simulink model "OFDM_Tx_Rx_fixed_point"  (R2020a)
settings: Solver=FixedStepDiscrete  StartTime=0.0  StopTime=inf  RelTol=1e-3
PostLoadFcn:
  | run ./scripts/filter_setup;
InitFcn:
  | % Set parameters
  | fs = 1e6;
  | 
  | % Load all required variables
  | load('variables/read_addr_data');
  | load('variables/read_addr_cp');
  | load('variables/read_addr_pream');
  | load('variables/read_addr_rx');
  | load('variables/pilot');
  | load('variables/sc_index');
  | load('variables/LTSfreq');
  | load('variables/STSfreq');
  | load('variables/LTSread');
  | load('variables/STSread');
undefined symbols (not defined in the file): CIC_fine_Rx, CIC_fine_Tx
libraries: dspmlti4 x7, OFDM_Rx x1, OFDM_Tx x1, dspobslib x1
settings Model: SimulationMode=accelerator  Creator=njb13206  LastModifiedBy=LDM
settings OptimizationCC: BlockReduction=off  ConditionallyExecuteInputs=off  DefaultParameterBehavior=Inlined
settings DebuggingCC: AlgebraicLoopMsg=error  IntegerOverflowMsg=none  ParameterPrecisionLossMsg=none  IntegerSaturationMsg=none
settings HardwareCC: ProdBitPerPointer=32  ProdBitPerSizeT=32  ProdBitPerPtrDiffT=32  ProdLargestAtomicFloat=None  ProdIntDivRoundTo=Undefined  ProdEndianess=Unspecified  ProdWordSize=32  ProdHWDeviceType=ASIC/FPGA->ASIC/FPGA  TargetBitPerPointer=64  TargetBitPerSizeT=64  TargetBitPerPtrDiffT=64  TargetLongLongMode=on  TargetIntDivRoundTo=Zero  TargetEndianess=LittleEndian  TargetWordSize=64  TargetHWDeviceType=Custom Processor->MATLAB Host Computer  ProdEqTarget=off

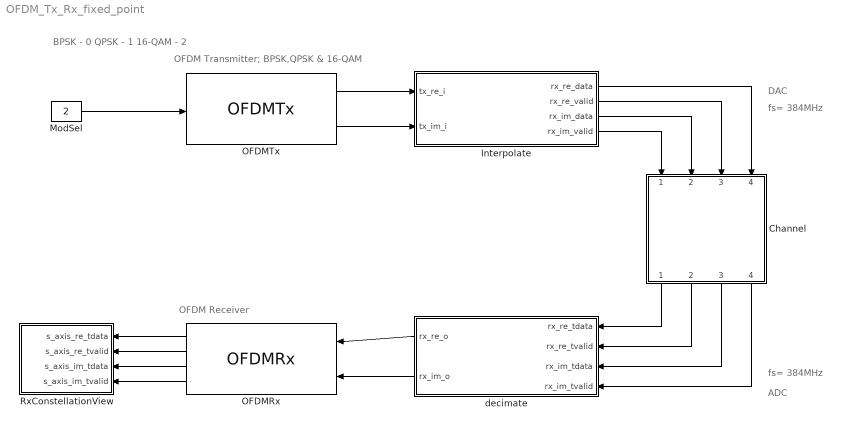
== system OFDM_Tx_Rx_fixed_point ==
  note: DAC
  note: OFDM Receiver
  note: OFDM Transmitter; BPSK,QPSK & 16-QAM
  note: BPSK - 0
      | QPSK - 1
      | 16-QAM - 2
  note: fs= 384MHz
  note: ADC
  note: fs= 384MHz
  "Channel " : Subsystem
  Interpolate : Subsystem
  ModSel : Constant  Value=2  OutDataTypeStr=fixdt(0,2,0)  SampleTime=1/fs
  OFDMRx : OFDM_Rx/OFDMRx  SystemSampleTime=-1  Latency=0  AutoFrameSizeCalculation=off
  OFDMTx : OFDM_Tx/OFDMTx  SystemSampleTime=-1  Latency=0  AutoFrameSizeCalculation=off
  RxConstellationView : Subsystem
  decimate : Subsystem
  wires:
  OFDMRx/1 -> RxConstellationView/1(s_axis_re_tdata)
  OFDMRx/2 -> RxConstellationView/2(s_axis_re_tvalid)
  ModSel/1 -> OFDMTx/1
  OFDMTx/1 -> Interpolate/1(tx_re_i)
  decimate/1(rx_re_o) -> OFDMRx/1
  OFDMTx/2 -> Interpolate/2(tx_im_i)
  decimate/2(rx_im_o) -> OFDMRx/2
  OFDMRx/3 -> RxConstellationView/3(s_axis_im_tdata)
  OFDMRx/4 -> RxConstellationView/4(s_axis_im_tvalid)
  "Channel "/1(chanOut_re) -> decimate/1(rx_re_tdata)
  "Channel "/2(tvalid_re_out) -> decimate/2(rx_re_tvalid)
  "Channel "/3(chanOut_im) -> decimate/3(rx_im_tdata)
  "Channel "/4(tvalid_im_out) -> decimate/4(rx_im_tvalid)
  Interpolate/1(rx_re_data) -> "Channel "/4(chanIn_re)
  Interpolate/2(rx_re_valid) -> "Channel "/3(m_re_tvalid)
  Interpolate/3(rx_im_data) -> "Channel "/2(chanIn_im)
  Interpolate/4(rx_im_valid) -> "Channel "/1(m_im_tvalid)

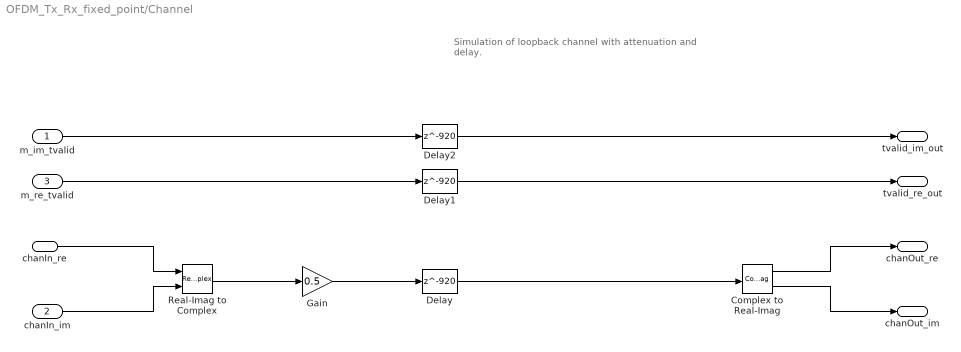
== system OFDM_Tx_Rx_fixed_point/Channel  ==
  note: Simulation of loopback channel with attenuation and
      | delay.
  m_im_tvalid : Inport
  chanIn_im : Inport  Port=2
  m_re_tvalid : Inport  Port=3
  chanIn_re : Inport  Port=4
  Complex to Real-Imag : ComplexToRealImag
  Delay : Delay  DelayLength=920
  Delay1 : Delay  DelayLength=920
  Delay2 : Delay  DelayLength=920
  Gain : Gain  Gain=0.5  ParamDataTypeStr=double  OutDataTypeStr=fixdt(1,16,14)
  Real-Imag to Complex : RealImagToComplex
  chanOut_re : Outport  VectorParamsAs1DForOutWhenUnconnected=off
  tvalid_re_out : Outport  Port=2  VectorParamsAs1DForOutWhenUnconnected=off
  chanOut_im : Outport  Port=3  VectorParamsAs1DForOutWhenUnconnected=off
  tvalid_im_out : Outport  Port=4  VectorParamsAs1DForOutWhenUnconnected=off
  wires:
  Delay2/1 -> tvalid_im_out/1
  Delay1/1 -> tvalid_re_out/1
  Complex to Real-Imag/2 -> chanOut_im/1
  Complex to Real-Imag/1 -> chanOut_re/1
  m_im_tvalid/1 -> Delay2/1
  m_re_tvalid/1 -> Delay1/1
  chanIn_im/1 -> Real-Imag to Complex/2
  chanIn_re/1 -> Real-Imag to Complex/1
  Real-Imag to Complex/1 -> Gain/1
  Gain/1 -> Delay/1
  Delay/1 -> Complex to Real-Imag/1

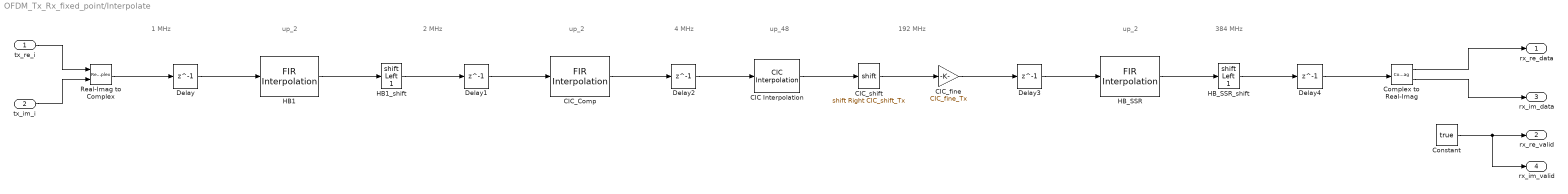
== system OFDM_Tx_Rx_fixed_point/Interpolate ==
  note: up_2
  note: 4 MHz
  note: 2 MHz
  note: 1 MHz
  note: 384 MHz
  note: 192 MHz
  note: up_2
  note: up_48
  note: up_2
  tx_re_i : Inport
  tx_im_i : Inport  Port=2
  CIC Interpolation : dspmlti4/CIC Interpolation  filtFrom=Filter object  filtobj=CIC  ftype=Interpolator  R=240  M=1  N=5  filterInternals=Full precision  BPS=[16 16 16 16]  FLPS=0  outputWordLength=32  outputFracLength=0  launchFVT=off  framing=Allow multirate processing  OutputFrames=off
      settings: SourceProductBaseCode=DS
  CIC_Comp : dspmlti4/FIR Interpolation  FilterSource=Dialog parameters  PrivateCoeffs=0  h=WComp.Numerator  L=2  FilterObject=FINTERP  framing=Allow multirate processing  outputBufInitCond=0  roundingMode=Floor  overflowMode=off  firstCoeffMode=Binary point scaling  firstCoeffWordLength=16  firstCoeffFracLength=15  firstCoeffDataTypeStr=fixdt(1,16,15)  firstCoeffMin=[]  firstCoeffMax=[]  firstCoeffLastDataTypeStr=fixdt(1,16,15)  outputMode=Binary point scaling  outputWordLength=16  outputFracLength=14  outputDataTypeStr=fixdt(1,16,14)  outputMin=[]  outputMax=[]  outputLastDataTypeStr=fixdt(1,16,14)
  CIC_fine : Gain  Gain=CIC_fine_Tx  OutDataTypeStr=fixdt(1,16,14)
  CIC_shift : ArithShift  BitShiftNumber=CIC_shift_Tx  BitShiftDirection=Right
  Complex to Real-Imag : ComplexToRealImag
  Constant : Constant  Value=true  SampleTime=1/384e6
  Delay{,1..4} (5 alike) : Delay  DelayLength=1
  HB1 : dspmlti4/FIR Interpolation  FilterSource=Dialog parameters  PrivateCoeffs=0  h=W_HB.Numerator  L=2  FilterObject=FINTERP  framing=Allow multirate processing  outputBufInitCond=0  roundingMode=Floor  overflowMode=off  firstCoeffMode=Binary point scaling  firstCoeffWordLength=16  firstCoeffFracLength=15  firstCoeffDataTypeStr=fixdt(1,16,15)  firstCoeffMin=[]  firstCoeffMax=[]  firstCoeffLastDataTypeStr=fixdt(1,16,15)  outputMode=Binary point scaling  outputWordLength=16  outputFracLength=14  outputDataTypeStr=fixdt(1,16,14)  outputMin=[]  outputMax=[]  outputLastDataTypeStr=fixdt(1,16,14)
  HB1_shift : ArithShift  BitShiftNumber=1  BitShiftDirection=Left
  HB_SSR : dspmlti4/FIR Interpolation  FilterSource=Dialog parameters  PrivateCoeffs=0  h=W_HB_ssr.Numerator  L=2  FilterObject=FINTERP  framing=Allow multirate processing  outputBufInitCond=0  roundingMode=Floor  overflowMode=off  firstCoeffMode=Binary point scaling  firstCoeffWordLength=16  firstCoeffFracLength=15  firstCoeffDataTypeStr=fixdt(1,16,15)  firstCoeffMin=[]  firstCoeffMax=[]  firstCoeffLastDataTypeStr=fixdt(1,16,15)  outputMode=Binary point scaling  outputWordLength=16  outputFracLength=14  outputDataTypeStr=fixdt(1,16,14)  outputMin=[]  outputMax=[]  outputLastDataTypeStr=fixdt(1,16,14)
  HB_SSR_shift : ArithShift  BitShiftNumber=1  BitShiftDirection=Left
  Real-Imag to Complex : RealImagToComplex
  rx_re_data : Outport
  rx_re_valid : Outport  Port=2
  rx_im_data : Outport  Port=3
  rx_im_valid : Outport  Port=4
  wires:
  CIC_fine/1 -> Delay3/1
  CIC_shift/1 -> CIC_fine/1
  HB_SSR_shift/1 -> Delay4/1
  HB_SSR/1 -> HB_SSR_shift/1
  CIC Interpolation/1 -> CIC_shift/1
  HB1_shift/1 -> Delay1/1
  CIC_Comp/1 -> Delay2/1
  HB1/1 -> HB1_shift/1
  Real-Imag to Complex/1 -> Delay/1
  tx_re_i/1 -> Real-Imag to Complex/1
  tx_im_i/1 -> Real-Imag to Complex/2
  Delay/1 -> HB1/1
  Delay1/1 -> CIC_Comp/1
  Delay2/1 -> CIC Interpolation/1
  Delay3/1 -> HB_SSR/1
  Delay4/1 -> Complex to Real-Imag/1
  Complex to Real-Imag/1 -> rx_re_data/1
  Complex to Real-Imag/2 -> rx_im_data/1
  Constant/1 -> rx_im_valid/1, rx_re_valid/1

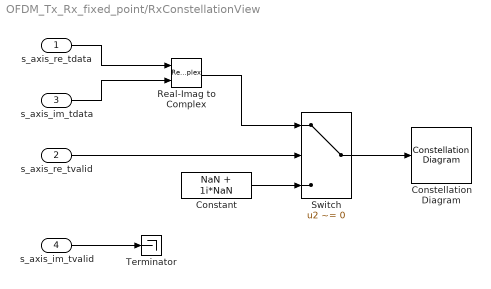
== system OFDM_Tx_Rx_fixed_point/RxConstellationView ==
  s_axis_re_tdata : Inport
  s_axis_re_tvalid : Inport  Port=2
  s_axis_im_tdata : Inport  Port=3
  s_axis_im_tvalid : Inport  Port=4
  Constant : Constant  Value=NaN + 1i*NaN  OutDataTypeStr=double  SampleTime=-1
  Constellation Diagram : ConstellationDiagram
  Real-Imag to Complex : RealImagToComplex
  Switch : Switch  Criteria=u2 ~= 0
  Terminator : Terminator
  wires:
  s_axis_im_tdata/1 -> Real-Imag to Complex/2
  s_axis_re_tdata/1 -> Real-Imag to Complex/1
  s_axis_im_tvalid/1 -> Terminator/1
  Real-Imag to Complex/1 -> Switch/1
  s_axis_re_tvalid/1 -> Switch/2
  Constant/1 -> Switch/3
  Switch/1 -> Constellation Diagram/1

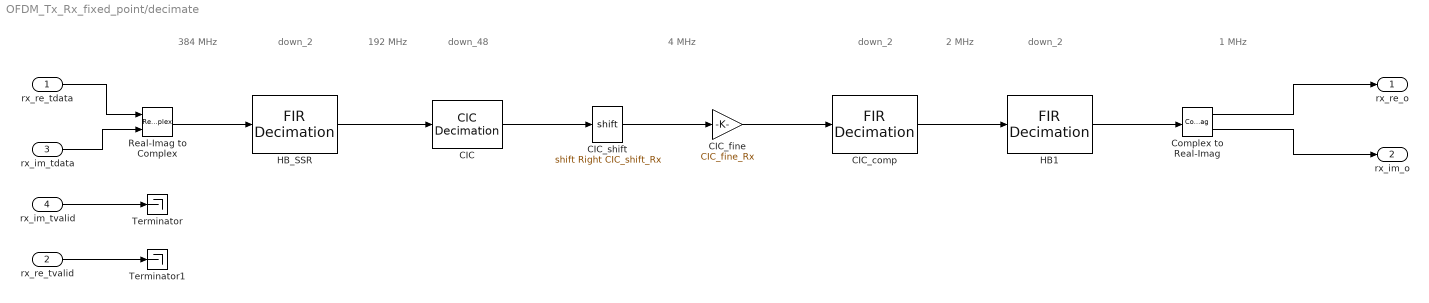
== system OFDM_Tx_Rx_fixed_point/decimate ==
  note: down_2
  note: down_2
  note: down_48
  note: 1 MHz
  note: 384 MHz
  note: 192 MHz
  note: 4 MHz
  note: 2 MHz
  note: down_2
  rx_re_tdata : Inport
  rx_re_tvalid : Inport  Port=2
  rx_im_tdata : Inport  Port=3
  rx_im_tvalid : Inport  Port=4
  CIC : dspobslib/CIC Decimation  filtFrom=Multirate object in workspace  filtobj=CIC_Rx  ftype=Decimator  R=2  M=1  N=2  filterInternals=Full precision  BPS=[16 16 16 16]  FLPS=0  outputWordLength=32  outputFracLength=0  launchFVT=off  framing=Maintain input frame rate  RateOptions=Allow multirate processing
      settings: SourceProductBaseCode=DS
  CIC_comp : dspmlti4/FIR Decimation  FilterSource=Dialog parameters  h=WComp_Rx.Numerator  D=2  filtStruct=Direct form  FilterObject=FDECIM  framing=Allow multirate processing  inputOffset=0  outputBufInitCond=0  roundingMode=Floor  overflowMode=off  firstCoeffMode=Binary point scaling  firstCoeffWordLength=16  firstCoeffFracLength=15  firstCoeffDataTypeStr=fixdt(1,16,15)  firstCoeffMin=[]  firstCoeffMax=[]  firstCoeffLastDataTypeStr=fixdt(1,16,15)  outputMode=Binary point scaling  outputWordLength=16  outputFracLength=14  outputDataTypeStr=fixdt(1,16,14)  outputMin=[]  outputMax=[]  outputLastDataTypeStr=fixdt(1,16,14)
  CIC_fine : Gain  Gain=CIC_fine_Rx  OutDataTypeStr=fixdt(1,16,14)
  CIC_shift : ArithShift  BitShiftNumber=CIC_shift_Rx  BitShiftDirection=Right
  Complex to Real-Imag : ComplexToRealImag
  HB1 : dspmlti4/FIR Decimation  FilterSource=Dialog parameters  h=W_HB.Numerator  D=2  filtStruct=Direct form  FilterObject=FDECIM  framing=Allow multirate processing  inputOffset=0  outputBufInitCond=0  roundingMode=Floor  overflowMode=off  firstCoeffMode=Binary point scaling  firstCoeffWordLength=16  firstCoeffFracLength=15  firstCoeffDataTypeStr=fixdt(1,16,15)  firstCoeffMin=[]  firstCoeffMax=[]  firstCoeffLastDataTypeStr=fixdt(1,16,15)  outputMode=Binary point scaling  outputWordLength=16  outputFracLength=14  outputDataTypeStr=fixdt(1,16,14)  outputMin=[]  outputMax=[]  outputLastDataTypeStr=fixdt(1,16,14)
  HB_SSR : dspmlti4/FIR Decimation  FilterSource=Dialog parameters  h=W_HB.Numerator  D=2  filtStruct=Direct form  FilterObject=FDECIM  framing=Allow multirate processing  inputOffset=0  outputBufInitCond=0  roundingMode=Floor  overflowMode=off  firstCoeffMode=Binary point scaling  firstCoeffWordLength=16  firstCoeffFracLength=15  firstCoeffDataTypeStr=fixdt(1,16,15)  firstCoeffMin=[]  firstCoeffMax=[]  firstCoeffLastDataTypeStr=fixdt(1,16,15)  outputMode=Binary point scaling  outputWordLength=16  outputFracLength=14  outputDataTypeStr=fixdt(1,16,14)  outputMin=[]  outputMax=[]  outputLastDataTypeStr=fixdt(1,16,14)
  Real-Imag to Complex : RealImagToComplex
  Terminator : Terminator
  Terminator1 : Terminator
  rx_re_o : Outport
  rx_im_o : Outport  Port=2
  wires:
  rx_re_tvalid/1 -> Terminator1/1
  rx_im_tvalid/1 -> Terminator/1
  Real-Imag to Complex/1 -> HB_SSR/1
  Complex to Real-Imag/2 -> rx_im_o/1
  Complex to Real-Imag/1 -> rx_re_o/1
  HB1/1 -> Complex to Real-Imag/1
  CIC_fine/1 -> CIC_comp/1
  CIC/1 -> CIC_shift/1
  HB_SSR/1 -> CIC/1
  CIC_shift/1 -> CIC_fine/1
  CIC_comp/1 -> HB1/1
  rx_re_tdata/1 -> Real-Imag to Complex/1
  rx_im_tdata/1 -> Real-Imag to Complex/2
